simulink model "rebi_multivariable"  (Simulink 7.6)
settings: Solver=ode1  StartTime=0.0  StopTime=50  FixedStep=0.001  RelTol=1e-3
PostLoadFcn:
  | , if any(exist('dsrtsu_mdlpostloadfcn', 'file') == [2, 3, 6]), try dsrtsu_mdlpostloadfcn('Execute', bdroot); catch fprintf('Error in PostLoadFcn (dsrtsu_mdlpostloadfcn) for model "%s":\n %s\n', bdroot, lasterr); end, end,
values from neighbouring files (symbols this model uses):
  A = [0 1 0 0 0 ... (first row only)    [vars_ed2.m]
  B = [0 0 ... (first row only)    [vars_ed2.m]
  C = [ 1 0 0 0 0 ... (first row only)    [vars_ed2.m]
  Ki = K(:,n+1:n+p)    [vars_ed2.m]
  Kp = K(:,1:n)    [vars_ed2.m]
settings Model: DSRTSU_INTERNAL_RTI_VER=370  DSRTSU_INTERNAL_RTI_TYPE=rti1104  Creator=eleve  LastModifiedBy=eleve  BufferReuse=off
settings OptimizationCC: BlockReduction=off  OptimizeBlockIOStorage=off  BufferReuse=off  ExpressionFolding=off  LocalBlockOutputs=off
settings HardwareCC: ProdIntDivRoundTo=Zero  ProdEndianess=BigEndian  ProdHWDeviceType=Generic->Custom  TargetIntDivRoundTo=Zero  TargetEndianess=BigEndian  TargetHWDeviceType=Generic->Custom
settings RTWCC: SystemTargetFile=rti1104.tlc  MakeCommand=make_rti  TemplateMakefile=rti1104.tmf  Description=dSPACE DS1104 Hardware Platform  ProcessScript=rti1104_make_rtw_hook
settings STFCustomTargetCC: ParMdlRefBuildCompliant=on  GeneratePreprocessorConditionals=Disable all  SystemTargetFile=rti1104.tlc
settings GRTTargetCC: CompOptLevelCompliant=off  MatFileLogging=off  ExtModeMexFile=noextcomm
settings CustomProperty: DataType=RTWOptions_EnumType_C__dSPACE_matlab_rti1104_tlc_rti1104_1InitialSimState  Value=RUN
settings EnumStrPairs: String=RUN

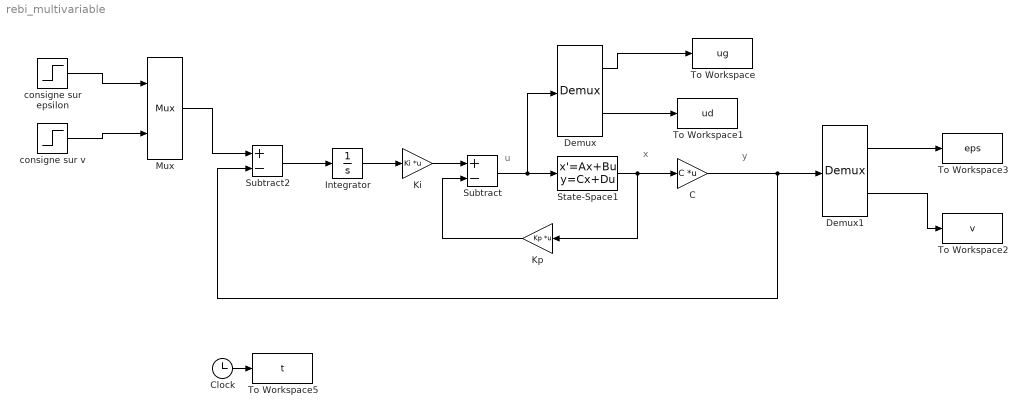
== system rebi_multivariable ==
  note: u
  note: x
  note: y
  C : Gain  Gain=C  Multiplication=Matrix(K*u) (u vector)
  Clock : Clock
      settings: Decimation=10
  Demux : Demux  Outputs=2
  Demux1 : Demux  Outputs=2
  Integrator : Integrator
  Ki : Gain  Gain=Ki  Multiplication=Matrix(K*u) (u vector)
  Kp : Gain  Gain=Kp  Multiplication=Matrix(K*u) (u vector)
  Mux : Mux  Inputs=2
  State-Space1 : StateSpace  A=A  B=B  C=eye(5)  D=zeros(5,2)
  Subtract : Sum  Inputs=+-
  Subtract2 : Sum  Inputs=+-
  To Workspace : ToWorkspace  VariableName=ug  SampleTime=-1  SaveFormat=Array
  To Workspace1 : ToWorkspace  VariableName=ud  SampleTime=-1  SaveFormat=Array
  To Workspace2 : ToWorkspace  VariableName=v  SampleTime=-1  SaveFormat=Array
  To Workspace3 : ToWorkspace  VariableName=eps  SampleTime=-1  SaveFormat=Array
  To Workspace5 : ToWorkspace  VariableName=t  SampleTime=-1  SaveFormat=Array
  consigne sur epsilon : Step  Time=6  After=pi/6  SampleTime=0
  consigne sur v : Step  Time=6  SampleTime=0
  wires:
  Subtract2/1 -> Integrator/1
  Integrator/1 -> Ki/1
  Ki/1 -> Subtract/1
  Kp/1 -> Subtract/2
  Subtract/1 -> State-Space1/1, Demux/1
  State-Space1/1 -> Kp/1, C/1
  C/1 -> Subtract2/2, Demux1/1
  consigne sur epsilon/1 -> Mux/1
  consigne sur v/1 -> Mux/2
  Mux/1 -> Subtract2/1
  Demux/1 -> To Workspace/1
  Demux/2 -> To Workspace1/1
  Demux1/1 -> To Workspace3/1
  Demux1/2 -> To Workspace2/1
  Clock/1 -> To Workspace5/1
